simulink model "PID_Controller"  (R2019b)
settings: Solver=VariableStepAuto  StartTime=0.0  StopTime=10  RelTol=1e-6
values from neighbouring files (symbols this model uses):
  A = [0 1; -2 3]    [Kalman_FSFB.m]    (also in LQR_MSD.m = [0      1)
  B = [0 1]'    [Kalman_FSFB.m]    (also in LQR_MSD.m = [0)
  C = [1 1]    [Kalman_FSFB.m]    (also in LQR_MSD.m = eye(2))
  D = [1]    [Kalman_FSFB.m]    (also in LQR_MSD.m = [0)
settings Model: Creator=bala4krish  LastModifiedBy=bala4krish

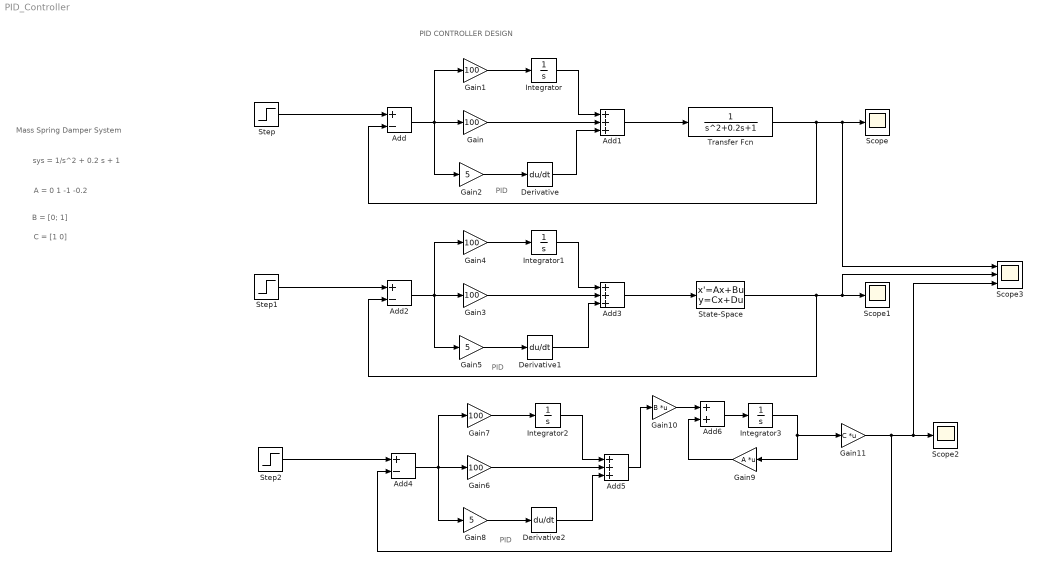
== system PID_Controller ==
  note: PID CONTROLLER DESIGN
  note: PID
  note: PID
  note: PID
  note: B = [0; 1]
  note: sys = 1/s^2 + 0.2 s + 1
  note: Mass Spring Damper System
  note: A =   0     1
      | 	-1   -0.2
  note: C = [1 0]
  Add : Sum  Inputs=+-
  Add1 : Sum  Inputs=+++
  Add2 : Sum  Inputs=+-
  Add3 : Sum  Inputs=+++
  Add4 : Sum  Inputs=+-
  Add5 : Sum  Inputs=+++
  Add6 : Sum
  Derivative : Derivative
  Derivative1 : Derivative
  Derivative2 : Derivative
  Gain{,1,3..4,6..7} (6 alike) : Gain  Gain=100
  Gain10 : Gain  Gain=B  Multiplication=Matrix(K*u)
  Gain11 : Gain  Gain=C  Multiplication=Matrix(K*u)
  Gain2 : Gain  Gain=5
  Gain5 : Gain  Gain=5
  Gain8 : Gain  Gain=5
  Gain9 : Gain  Gain=A  Multiplication=Matrix(K*u)
  Integrator : Integrator  InitialCondition=1
  Integrator1 : Integrator  InitialCondition=1
  Integrator2 : Integrator  InitialCondition=1
  Integrator3 : Integrator
  Scope : Scope
  Scope1 : Scope
  Scope2 : Scope
  Scope3 : Scope  NumInputPorts=3
  State-Space : StateSpace  A=A  B=B  C=C  D=D  InitialCondition=0
  Step : Step  Time=0  SampleTime=0
  Step1 : Step  Time=0  SampleTime=0
  Step2 : Step  Time=0  SampleTime=0
  Transfer Fcn : TransferFcn  Denominator=[1 0.2 1]
  wires:
  Transfer Fcn/1 -> Add/2, Scope3/1, Scope/1
  Add/1 -> Gain2/1, Gain1/1, Gain/1
  Step/1 -> Add/1
  Gain1/1 -> Integrator/1
  Integrator/1 -> Add1/1
  Gain/1 -> Add1/2
  Gain2/1 -> Derivative/1
  Derivative/1 -> Add1/3
  Add1/1 -> Transfer Fcn/1
  Add2/1 -> Gain5/1, Gain4/1, Gain3/1
  Integrator1/1 -> Add3/1
  Gain5/1 -> Derivative1/1
  Derivative1/1 -> Add3/3
  Step1/1 -> Add2/1
  State-Space/1 -> Add2/2, Scope3/2, Scope1/1
  Gain3/1 -> Add3/2
  Gain4/1 -> Integrator1/1
  Add3/1 -> State-Space/1
  Gain6/1 -> Add5/2
  Add4/1 -> Gain8/1, Gain7/1, Gain6/1
  Gain7/1 -> Integrator2/1
  Gain8/1 -> Derivative2/1
  Integrator2/1 -> Add5/1
  Step2/1 -> Add4/1
  Derivative2/1 -> Add5/3
  Integrator3/1 -> Gain11/1, Gain9/1
  Gain10/1 -> Add6/1
  Add5/1 -> Gain10/1
  Gain9/1 -> Add6/2
  Add6/1 -> Integrator3/1
  Gain11/1 -> Add4/2, Scope3/3, Scope2/1
